simulink model "Katex_FullCar_R2017b_V03"  (R2026a)
settings: Solver=ode1  StopTime=1000  FixedStep=Ts  EnableMultiTasking=on
PostLoadFcn:
  | , if any(exist('dsrtsu_mdlpostloadfcn', 'file') == [2, 3, 6]), try dsrtsu_mdlpostloadfcn('Execute', bdroot); catch fprintf('Error in PostLoadFcn (dsrtsu_mdlpostloadfcn) for model "%s":\n %s\n', bdroot, lasterr); end, end,
  | , if any(exist('dsrtsu_mdlpostloadfcn', 'file') ~= 0), dsrtsu_mdlpostloadfcn('Execute', bdroot); end,
InitFcn:
  | , if any(exist('rtifpga_mdlclblib', 'file') ~= 0), rtifpga_mdlclblib('Init', bdroot); end,
  | 
  | 
  | init
undefined symbols (not defined in the file): locklim_sus, roundN, Ts
libraries: sl_discontinuities x29, simulink_extras x26, simulink x22, mjLib x1
(part 1 of 10)
Description:
  | Standard RTI1401 template.
  | Supported MATLAB version:  R2018b.
settings Model: Tag=RTI1401  DSRTSU_INTERNAL_RTI_VER=510  DSRTSU_INTERNAL_RTI_TYPE=rti1401  RTICANMMDATA=struct('GeneralSetupData',struct('modelroot','C:\Users\USER\Desktop\KATEC_FullCar\simulink','generalsettings',struct('filesettings',struct('destfolder',struct('Name','RTICANMM_FILES','Check',1),'buildfolder',struct('Name','.','Check',1),'AbsDestfolder',struct('Name','C:\Users\USER\Desktop\KATEC_FullCar\simulink\RTICANMM_FILES'),'AbsBuildfolder',struct('Name','C:\Users\USER\Desktop\KATEC_FullCar\simulink'))),'options',struct('addpaths',1,'rmpaths',1,'addtrcexclusion',logical(1),'cannavigator',struct('checkmonitoring',0),'show_usrtrc',0,'use_usrtrc',0),'advanced',struct('options',[1 1 1 1 1 1 1 1 1 1 1 1 1 1 1 1 1 1 1 1 1 1 1 1 1 1 1 1 1 1 1 1 1 1 1 1 1 1 1 1 1 1 1 1 1 1 1 1 1 1 1 1 1 1 1 1 1 1 1 1 1 1 1 1 1 1 1 1 1 1 1 1 1 1 1 1 1 1 1 1 1 1 1 1 1 1 1 1 1 1 1 1 1 1 1 1 1 1 1 1]),'MPSetup',{{}},'modelname','Katex_FullCar_R2017b_V03','block','Katex_FullCar_R2017b_V03'))  DSRTSU_INTERNAL_RTIFLEXRAYCONFIG=110  DSRTSU_INTERNAL_RTIFPGA=110  Creator=KATECH  LastModifiedBy=minsu
settings DataIOCC: SaveFormat=StructureWithTime
settings OptimizationCC: OptimizeBlockIOStorage=off  BufferReuse=off  GlobalBufferReuse=off  ExpressionFolding=off  LocalBlockOutputs=off  OptimizeDataStoreBuffers=off  BusAssignmentInplaceUpdate=off
settings HardwareCC: ProdLargestAtomicInteger=Integer  ProdEndianess=BigEndian  ProdHWDeviceType=Custom Processor->Custom  TargetIntDivRoundTo=Zero  TargetEndianess=BigEndian  TargetHWDeviceType=Custom Processor->Custom
settings ModelReferenceCC: EnableParallelModelReferenceBuilds=on  ParallelModelReferenceMATLABWorkerInit=Load Top Model
settings RTWCC: SystemTargetFile=rti1401.tlc  MakeCommand=make_rti  TemplateMakefile=rti1401.tmf  RTWCompilerOptimization=on  Description=dSPACE DS1401 Hardware Platform
settings STFCustomTargetCC: SystemTargetFile=rti1401.tlc  MultiwordLength=2048.0  ParMdlRefBuildCompliant=on  GRTInterface=off  TRCGenerateLabels=off  AssertionMode=OFF  EnableDataSetStorageNonUI=OFF  TRCGenerateVirtualBlocks=off  TimeScaleFactorNonUI=OPTION_DISABLED  PlatformSelectionPopup=Platform Name  LoadAfterBuild=on  AllowReservedHostServiceNums=off  TRCGenerateParamValues=off  TRCGenerateStates=off  EnableRealTimeTestingNonUI=ON  LoadToFlash=off  CCompilerOptimizationOptsNonUI=USE_DEFAULT  NetworkClientNonUI=OPTION_DISABLED  EnableDataSetStorage=off  InitialSimState=RUN  ExecutionModeNonUI=RTSIM  LoadApplNonUI=ON  BoardName=ds1401  CCompilerOptimizationOptsPopup_=Default  TRCIsOmitVdOn=off  BoardNameNonUI=ds1401  TRCGenerateDerivatives=off  ExecutionMode=real-time  RTICfgSetVer=510.0  TimeScaleFactor=1.0  TRCOnlyGlobals=off  EnableRealTimeTesting=on
settings GRTTargetCC: CompOptLevelCompliant=off  ConcurrentExecutionCompliant=off  CombineOutputUpdateFcns=off  MatFileLogging=off  CPPClassGenCompliant=off
settings ConfigComp: CovMetricSettings=dswe
settings SimscapeCC: SimscapeLogDecimation=1  SimscapeLogType=none  SimscapeNominalValues="[{\"value\":\"1\",\"unit\":\"A\"},{\"value\":\"1\",\"unit\":\"bar\"},{\"value\":\"1\",\"unit\":\"cm^2\"},{\"value\":\"1\",\"unit\":\"cm^3/s\"},{\"value\":\"1\",\"unit\":\"kJ/kg\"},{\"value\":\"1\",\"unit\":\"kW\"},{\"value\":\"1\",\"unit\":\"l\"},{\"value\":\"1\",\"unit\":\"N\"},{\"value\":\"1\",\"unit\":\"N*m\"},{\"value\":\"1\",\"unit\":\"V\"}]"  SimscapeLogDataHistory=5000

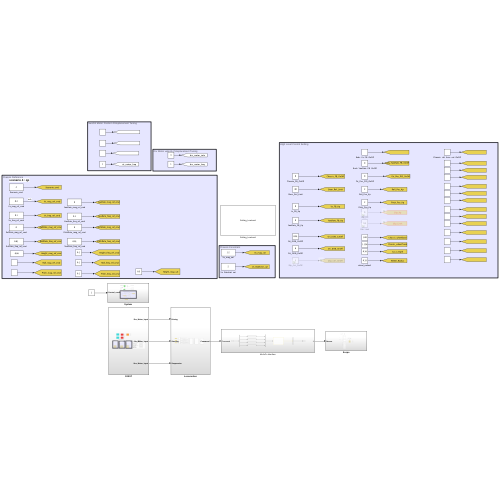
[thumbnail: Simulink's stored preview of the top-level diagram]
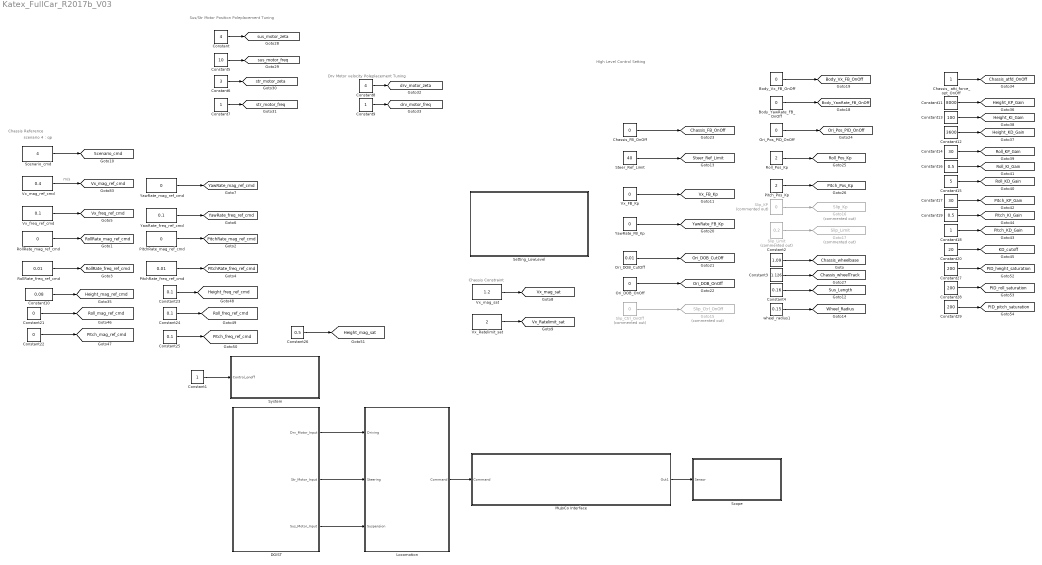
== system Katex_FullCar_R2017b_V03 ==
  note: scenario 4 : qp
  note: Chassis Reference
  note: Drv Motor velocity Poleplacement Tuning
  note: m/s
  note: Chassis Constraint
  note: HIgh Level Control Setting
  note: Sus/Str Motor Position Poleplacement Tuning
  Body_Vx_FB_OnOff : Constant  Value=0
  Body_YawRate_FB_OnOff : Constant  Value=0
  Chassis_ atti_force_opt_OnOff : Constant
  Chassis_FB_OnOff : Constant  Value=0
  Constant : Constant  Value=4
  Constant{1,7,9,18} (4 alike) : Constant
  Constant10 : Constant  Value=0.08
  Constant11 : Constant  Value=8000
  Constant12 : Constant  Value=3600
  Constant13 : Constant  Value=100
  Constant14 : Constant  Value=30
  Constant15 : Constant  Value=5
  Constant16 : Constant  Value=0.5
  Constant17 : Constant  Value=30
  Constant19 : Constant  Value=0.5
  Constant2 : Constant  Value=1.09
  Constant20 : Constant  Value=20
  Constant21 : Constant  Value=0
  Constant22 : Constant  Value=0
  Constant23 : Constant  Value=0.1
  Constant24 : Constant  Value=0.1
  Constant25 : Constant  Value=0.1
  Constant26 : Constant  Value=0.5
  Constant27 : Constant  Value=200
  Constant28 : Constant  Value=200
  Constant29 : Constant  Value=200
  Constant3 : Constant  Value=1.126
  Constant4 : Constant  Value=0.16
  Constant5 : Constant  Value=10
  Constant6 : Constant  Value=3
  Constant8 : Constant  Value=4
  DGIST : Subsystem
  Goto15 : Goto  Commented=on  GotoTag=Slip_Ctrl_OnOff  TagVisibility=global
  Goto16 : Goto  Commented=on  GotoTag=Slip_Kp  TagVisibility=global
  Goto17 : Goto  Commented=on  GotoTag=Slip_Limit  TagVisibility=global
  Locomotion : Subsystem
  MuJoCo Interface : Subsystem
  Ori_DOB_CutOff : Constant  Value=0.01
  Ori_DOB_OnOff : Constant  Value=0
  Ori_Pos_PID_OnOff : Constant  Value=0
  PitchRate_freq_ref_cmd : Constant  Value=0.01
  PitchRate_mag_ref_cmd : Constant  Value=0
  Pitch_Pos_Kp : Constant  Value=2
  RollRate_freq_ref_cmd : Constant  Value=0.01
  RollRate_mag_ref_cmd : Constant  Value=0
  Roll_Pos_Kp : Constant  Value=2
  Scenario_cmd : Constant  Value=4
  Scope : Subsystem
  Setting_LowLevel : Subsystem
      mask Display: disp('Setting_LowLevel');
  Slip_Ctrl_OnOff : Constant  Commented=on  Value=0
  Slip_KP : Constant  Commented=on  Value=0
  Slip_Limit : Constant  Commented=on  Value=0.2
  Steer_Ref_Limit : Constant  Value=40
  System : Subsystem
  Vx_FB_Kp : Constant  Value=0
  Vx_Ratelimit_sat : Constant  Value=2
  Vx_freq_ref_cmd : Constant  Value=0.1
  Vx_mag_ref_cmd : Constant  Value=0.4
  Vx_mag_sat : Constant  Value=1.2
  YawRate_FB_Kp : Constant  Value=0
  YawRate_freq_ref_cmd : Constant  Value=0.1
  YawRate_mag_ref_cmd : Constant  Value=0
  wheel_radius1 : Constant  Value=0.15
  tag scope: Body_Vx_FB_OnOff=global, Body_YawRate_FB_OnOff=global, Chassis_FB_OnOff=global, Chassis_atfd_OnOff=global, Chassis_wheelTrack=global, Chassis_wheelbase=global, Height_KD_Gain=global, Height_KI_Gain=global, Height_KP_Gain=global, Height_freq_ref_cmd=global, Height_mag_ref_cmd=global, Height_mag_sat=global, KD_cutoff=global, Ori_DOB_CutOff=global, Ori_DOB_OnOff=global, Ori_Pos_PID_OnOff=global, PID_height_saturation=global, PID_pitch_saturation=global, PID_roll_saturation=global, PitchRate_freq_ref_cmd=global, PitchRate_mag_ref_cmd=global, Pitch_KD_Gain=global, Pitch_KI_Gain=global, Pitch_KP_Gain=global, Pitch_Pos_Kp=global, Pitch_freq_ref_cmd=global, Pitch_mag_ref_cmd=global, RollRate_freq_ref_cmd=global, RollRate_mag_ref_cmd=global, Roll_KD_Gain=global, Roll_KI_Gain=global, Roll_KP_Gain=global, Roll_Pos_Kp=global, Roll_freq_ref_cmd=global, Roll_mag_ref_cmd=global, Scenario_cmd=global, Steer_Ref_Limit=global, Sus_Length=global, Vx_FB_Kp=global, Vx_Ratelimit_sat=global, Vx_freq_ref_cmd=global, Vx_mag_ref_cmd=global, Vx_mag_sat=global, Wheel_Radius=global, YawRate_FB_Kp=global, YawRate_freq_ref_cmd=global, YawRate_mag_ref_cmd=global, drv_motor_freq=global, drv_motor_zeta=global, str_motor_freq=global, str_motor_zeta=global, sus_motor_freq=global, sus_motor_zeta=global
  wires:
  DGIST/1(Drv_Motor_Input) -> Locomotion/1(Driving)
  DGIST/2(Str_Motor_Input) -> Locomotion/2(Steering)
  MuJoCo Interface/1(Out1) -> Scope/1(Sensor)
  Locomotion/1(Command) -> MuJoCo Interface/1(Command)
  Constant1/1 -> System/1(Control_onoff)
  RollRate_freq_ref_cmd/1 -> [RollRate_freq_ref_cmd]
  YawRate_freq_ref_cmd/1 -> [YawRate_freq_ref_cmd]
  Vx_mag_ref_cmd/1 -> [Vx_mag_ref_cmd]
  RollRate_mag_ref_cmd/1 -> [RollRate_mag_ref_cmd]
  Vx_Ratelimit_sat/1 -> [Vx_Ratelimit_sat]
  Vx_freq_ref_cmd/1 -> [Vx_freq_ref_cmd]
  Scenario_cmd/1 -> [Scenario_cmd]
  PitchRate_mag_ref_cmd/1 -> [PitchRate_mag_ref_cmd]
  Vx_mag_sat/1 -> [Vx_mag_sat]
  PitchRate_freq_ref_cmd/1 -> [PitchRate_freq_ref_cmd]
  YawRate_mag_ref_cmd/1 -> [YawRate_mag_ref_cmd]
  Constant2/1 -> [Chassis_wheelbase]
  Slip_Ctrl_OnOff/1 -> Goto15/1
  Body_YawRate_FB_OnOff/1 -> [Body_YawRate_FB_OnOff]
  Vx_FB_Kp/1 -> [Vx_FB_Kp]
  Ori_Pos_PID_OnOff/1 -> [Ori_Pos_PID_OnOff]
  Slip_KP/1 -> Goto16/1
  YawRate_FB_Kp/1 -> [YawRate_FB_Kp]
  Roll_Pos_Kp/1 -> [Roll_Pos_Kp]
  Pitch_Pos_Kp/1 -> [Pitch_Pos_Kp]
  Constant4/1 -> [Sus_Length]
  Slip_Limit/1 -> Goto17/1
  Ori_DOB_OnOff/1 -> [Ori_DOB_OnOff]
  Ori_DOB_CutOff/1 -> [Ori_DOB_CutOff]
  Steer_Ref_Limit/1 -> [Steer_Ref_Limit]
  Chassis_FB_OnOff/1 -> [Chassis_FB_OnOff]
  wheel_radius1/1 -> [Wheel_Radius]
  Body_Vx_FB_OnOff/1 -> [Body_Vx_FB_OnOff]
  Constant3/1 -> [Chassis_wheelTrack]
  Constant/1 -> [sus_motor_zeta]
  Constant5/1 -> [sus_motor_freq]
  Constant7/1 -> [str_motor_freq]
  Constant6/1 -> [str_motor_zeta]
  Constant8/1 -> [drv_motor_zeta]
  Constant9/1 -> [drv_motor_freq]
  Chassis_ atti_force_opt_OnOff/1 -> [Chassis_atfd_OnOff]
  DGIST/3(Sus_Motor_Input) -> Locomotion/3(Suspension)
  Constant11/1 -> [Height_KP_Gain]
  Constant12/1 -> [Height_KD_Gain]
  Constant13/1 -> [Height_KI_Gain]
  Constant14/1 -> [Roll_KP_Gain]
  Constant16/1 -> [Roll_KI_Gain]
  Constant15/1 -> [Roll_KD_Gain]
  Constant17/1 -> [Pitch_KP_Gain]
  Constant19/1 -> [Pitch_KI_Gain]
  Constant18/1 -> [Pitch_KD_Gain]
  Constant20/1 -> [KD_cutoff]
  Constant10/1 -> [Height_mag_ref_cmd]
  Constant21/1 -> [Roll_mag_ref_cmd]
  Constant22/1 -> [Pitch_mag_ref_cmd]
  Constant23/1 -> [Height_freq_ref_cmd]
  Constant24/1 -> [Roll_freq_ref_cmd]
  Constant25/1 -> [Pitch_freq_ref_cmd]
  Constant26/1 -> [Height_mag_sat]
  Constant27/1 -> [PID_height_saturation]
  Constant28/1 -> [PID_roll_saturation]
  Constant29/1 -> [PID_pitch_saturation]

== system Katex_FullCar_R2017b_V03/DGIST ==
  note: Str Plant Input
      |
      | Motor Input => cnt or Target Torque
  note: Plant Input에 연결시키면 됨
  note: Hardware ActVal에서 변환 필요
  note: Drive Plant Input
      |
      | Motor Input => RPM or Target Torque
  note: Motor Driver
      | vel은 RPM / Pos cnt / Torque mA로 나옴(모터 상수이용해서 Nm 교체 필요)
      | Dri__ , Sus__, Str__ , 빈칸에는 FL,FR,RL,RR 작성 필요
      | 각 Controller에 measure 자리에 집어 넣어야함
      |
      | Drive Wheel단 Load rad/s measure
      | Drive wheel단 Load Nm measure
      |
      | Suspension Load deg measure
      | Suspension Load rad/s measure
      | Suspension Load Nm measure
      | Suspension Load rad measure(highlevel)
      |
      | Steer Load deg measure
      | Steer Load Nm measure
      |
      | IMU RollRate LPF measure
      | IMU PitchRate LPF measure
      | IMU Roll angle LPF measure
      | IMU Pitch angle LPF measure
      |
      | 후륜 Load rad/s를 가지고 Vx setting
      | slip ratio도 해당꺼로 계산 필요
  note: Sus Plant Input
      |
      | Motor Input => cnt or RPM
      | Not Yet Torque Mode
  Attitude&Force distribution opt : Subsystem
      mask Display: disp('Force Distribution Opt');
  Attitude_reference_generator : Subsystem
      mask Display: disp('_Reference_Generator')
  Subsystem : Subsystem
      mask Display: disp('Dri_actRPM_2_Load[Rad/s]');
  Subsystem1 : Subsystem
      mask Display: disp('Dri_actTorque_2_Load[Nm]');
  Subsystem10 : Subsystem  Commented=on
      mask Display: disp('Imu_Pitch_LPF');
  Subsystem11 : Subsystem
      mask Display: disp('Sus_actPos_2_Load[rad]');
  Subsystem12 : Subsystem  Commented=on
      mask Display: disp('Imu_RollRate_LPF');
  Subsystem13 : Subsystem
      mask Display: disp('Dri_ref(m/s)_2_motor(rad/s)');
  Subsystem2 : Subsystem
      mask Display: disp('Sus_actPos_2_Load[deg]');
  Subsystem3 : Subsystem
      mask Display: disp('Sus_actVel_2_Load[rad/s]');
  Subsystem4 : Subsystem
      mask Display: disp('Sus_actTorque_2_Load[Nm]');
  Subsystem5 : Subsystem
      mask Display: disp('Str_actTorque_2_Load[Nm]');
  Subsystem6 : Subsystem
      mask Display: disp('Str_actPos_2_Load[deg]');
  Subsystem7 : Subsystem  Commented=on
      mask Display: disp('Imu_PitchRate_LPF');
  Subsystem8 : Subsystem  Commented=on
      mask Display: disp('Imu_RollRate_LPF');
  Subsystem9 : Subsystem  Commented=on
      mask Display: disp('Imu_Roll_LPF');
  _High_Level_Ctrl : Subsystem
      mask Display: disp('High Level Controller');
  _Low_Level_Ctrl : Subsystem
      mask Display: disp('Low Level Controller')
  _Reference_Generator : Subsystem
      mask Display: disp('_Reference_Generator')
  Drv_Motor_Input : Outport  VectorParamsAs1DForOutWhenUnconnected=off
  Str_Motor_Input : Outport  Port=2  VectorParamsAs1DForOutWhenUnconnected=off
  Sus_Motor_Input : Outport  Port=3  VectorParamsAs1DForOutWhenUnconnected=off
  wires:
  _High_Level_Ctrl/2(Str_Load_Vel_Ref) -> _Low_Level_Ctrl/2(In2)  "Str_Load_Vel_Ref"
  _Low_Level_Ctrl/2(Out2) -> Str_Motor_Input/1
  _Low_Level_Ctrl/1(Out1) -> Drv_Motor_Input/1
  _Low_Level_Ctrl/3(Out3) -> Sus_Motor_Input/1
  Attitude_reference_generator/1(Out1) -> Attitude&Force distribution opt/1(u)
  Attitude&Force distribution opt/2(Desired_sus_torque[4X1]) -> _Low_Level_Ctrl/3(In3)  "Sus_Torque_Ref"
  Attitude&Force distribution opt/1(vx[m/s]) -> _Low_Level_Ctrl/1(In1)

== system Katex_FullCar_R2017b_V03/Locomotion ==
  Driving : Inport
  Steering : Inport  Port=2
  Suspension : Inport  Port=3
  Branch : Subsystem
  Conditioning : Subsystem
  If Action Subsystem : Subsystem  TreatAsAtomicUnit=on
  If Action Subsystem1 : Subsystem  TreatAsAtomicUnit=on
  If Action Subsystem2 : Subsystem  TreatAsAtomicUnit=on
  If Action Subsystem3 : Subsystem  TreatAsAtomicUnit=on
  If Action Subsystem4 : Subsystem  TreatAsAtomicUnit=on
  If Action Subsystem5 : Subsystem  TreatAsAtomicUnit=on
  If1 : If  IfExpression=u1 == 1  ElseIfExpressions=u1 == 2
  If2 : If  IfExpression=u1 == 0||u1==1  ElseIfExpressions=u1 == 2
  If3 : If  IfExpression=u1 == 0||u1==1  ElseIfExpressions=u1 == 2
  Initialization : Subsystem
  Command : Outport  VectorParamsAs1DForOutWhenUnconnected=off
  wires:
  Branch/3(RL) -> Initialization/3(RLin)
  Branch/4(RR) -> Initialization/4(RRin)
  Branch/2(FR) -> Initialization/2(FRin)
  Conditioning/3(Str_angle) -> Branch/3(str_angref_deg)
  Conditioning/2(Drv_torque) -> Branch/2(drv_tqref_Nm)
  Conditioning/5(Sus_angle) -> Branch/5(sus_angref_deg)
  Conditioning/4(Str_torque) -> Branch/4(str_tqref_Nm)
  Conditioning/1(Drv_velocity) -> Branch/1(drv_velref_mps)
  Branch/1(FL) -> Initialization/1(FLin)
  Initialization/1(Controller) -> Command/1
  Driving/1 -> If Action Subsystem/1(In1), If Action Subsystem1/1(Driving)
  [Dri_Motor_Mode] -> If1/1
  If1/1 -> If Action Subsystem/Action
  If Action Subsystem/1(CMD_DRV_VELOCITY) -> Conditioning/1(CMD_DRV_VELOCITY)
  If Action Subsystem1/1(CMD_DRV_VELOCITY) -> Conditioning/2(CMD_DRV_TORQUE)
  If1/2 -> If Action Subsystem1/Action
  Steering/1 -> If Action Subsystem3/1(Driving), If Action Subsystem2/1(In1)
  If2/2 -> If Action Subsystem3/Action
  If2/1 -> If Action Subsystem2/Action
  If Action Subsystem2/1(CMD_DRV_VELOCITY) -> Conditioning/3(CMD_STR_ANGLE)
  If Action Subsystem3/1(CMD_DRV_VELOCITY) -> Conditioning/4(CMD_STR_TORQUE)
  [Str_Motor_Mode] -> If2/1
  If3/2 -> If Action Subsystem5/Action
  If3/1 -> If Action Subsystem4/Action
  [Sus_Motor_Mode] -> If3/1
  Suspension/1 -> If Action Subsystem5/1(Driving), If Action Subsystem4/1(Suspension)
  If Action Subsystem4/1(CMD_DRV_VELOCITY) -> Conditioning/5(CMD_SUS_ANGLE)
  If Action Subsystem5/1(CMD_DRV_VELOCITY) -> Conditioning/6(CMD_SUS_TORQUE)
  Conditioning/6(Sus_torque) -> Branch/6(sus_tqref_Nm)

== system Katex_FullCar_R2017b_V03/MuJoCo Interface ==
  Command : Inport
  Bus Creator : BusCreator  Inputs=4
  Bus Selector : BusSelector  OutputSignals=torque_sensor_FL,torque_sensor_FR,torque_sensor_RL,torque_sensor_RR,imu_acc,imu_gyro,trunk_vel,trunk_angvel,trunk_pos,trunk_ang,ENC_FL_sus,ENC_FL_steer,ENC_FL_drive,ENC_FR_sus,ENC_FR_steer,ENC_FR_drive,ENC_RL_sus,ENC_RL_steer,ENC_RL_drive,ENC_RR_sus,ENC_RR_steer,ENC_RR_drive,touch_FL,grf_seonsor_FL,touch_FR,grf_seonsor_FR,touch_RL,grf_seonsor_RL,touch_RR,grf_seonsor_RR,Vel_FL_sus,Vel_FR_sus,Vel_RL_sus,Vel_RR_sus,Vel_FL_steer,Vel_FR_steer,Vel_RL_steer,Vel_RR_steer,Vel_FL_drv,Vel_FR_drv,Vel_RL_drv,Vel_RR_drv,FL_sus_actuator_torque,FR_sus_actuator_torque,RL_sus_actuator_torque,RR_sus_actuator_torque  OutputAsBus=on
  Bus Selector1 : BusSelector  OutputSignals=FL,FR,RL,RR
  FL_Motor_Control : Subsystem
  FR_Motor_Control : Subsystem
  MuJoCo Plant : mjLib/MuJoCo Plant  controlBus=[]  sensorBus=mj_bus_sensor_7979902499018342666  controlLength=[]  sensorLength=[]  rgbLength=[]  depthLength=[]  sampleTime=0.001  xmlFileRel=/home/minsu/MuJoCo_Rover_CTRL/model/mcl_rover/scene_terrain.xml  xmlFile=/home/minsu/MuJoCo_Rover_CTRL/model/mcl_rover/scene_terrain.xml  renderingType=Global  vsync=off  visualFPS=60  zoomLevel=1  znear=0.03  zfar=150  cameraSampleTime=0.001  rgbOutOption=on  depthOutOption=on  controlInterfaceType=Vector
      settings: SourceProductName=MuJoCo Simulator
  RL_Motor_Control : Subsystem
  RR_Motor_Control : Subsystem
  Out1 : Outport
  wires:
  RL_Motor_Control/1(Out2) -> Bus Creator/3  "RL"
  RR_Motor_Control/1(Out2) -> Bus Creator/4  "RR"
  Bus Creator/1 -> MuJoCo Plant/1
  FR_Motor_Control/1(Out2) -> Bus Creator/2  "FR"
  Command/1 -> Bus Selector1/1
  Bus Selector1/1 -> FL_Motor_Control/1(In1)  "<FL>"
  Bus Selector1/2 -> FR_Motor_Control/1(In1)  "<FR>"
  Bus Selector1/3 -> RL_Motor_Control/1(In1)  "<RL>"
  Bus Selector1/4 -> RR_Motor_Control/1(In1)  "<RR>"
  MuJoCo Plant/1 -> Bus Selector/1
  Bus Selector/1 -> Out1/1
  FL_Motor_Control/1(Out2) -> Bus Creator/1  "FL"

== system Katex_FullCar_R2017b_V03/Scope ==
  Sensor : Inport
  Body_PitchRate_ref : Scope
      settings: DataLoggingVariableName=ScopeData4
  Body_RollRate_ref : Scope
      settings: DataLoggingVariableName=ScopeData3
  Body_Vx_ref : Scope
  Body_YawRate_ref : Scope
      settings: DataLoggingVariableName=ScopeData2
  Controlword_cmd : Scope
      settings: DataLoggingVariableName=ScopeData28
  Demux : Demux  Outputs=2
  FL : Subsystem
  FR : Subsystem
  IMU : Subsystem
  Initialization_Status : Subsystem
  NMT_NodeID : Scope
      settings: DataLoggingVariableName=ScopeData27
  NMT_cmd : Scope
  RL : Subsystem
  RR : Subsystem
  TOUCH : Subsystem
  Torque_sensor : Scope  NumInputPorts=4
      settings: ActiveDisplayYMinimum=-8.5141737367185648  ActiveDisplayYMaximum=2.7458236474698614  DataLoggingVariableName=ScopeData96
  Trunk : Subsystem
  wires:
  [NMT] -> Demux/1
  Sensor/1 -> RR/1(Plant), TOUCH/1(Sensor), Trunk/1(Sensor), IMU/1(In1), RL/1(Plant), FR/1(Plant), FL/1(Plant)
  [Controller] -> FL/2(Controller), FR/2(Controller), RL/2(Controller), RR/2(Controller)
  Demux/1 -> NMT_cmd/1
  Demux/2 -> NMT_NodeID/1
  [controlword_cmd] -> Controlword_cmd/1
  [Body_Pitch_deg_scope] -> Body_PitchRate_ref/1
  [Body_Roll_deg_scope] -> Body_RollRate_ref/1
  [Body_Yawrate_degps_scope] -> Body_YawRate_ref/1
  [Body_vx_mps_scope] -> Body_Vx_ref/1
  [RL_sus_torque] -> Torque_sensor/3  "RL"
  [RR_Sus_torque] -> Torque_sensor/4  "RR"
  [FR_sus_torque] -> Torque_sensor/2  "FR"
  [FL_sus_torque] -> Torque_sensor/1  "FL"

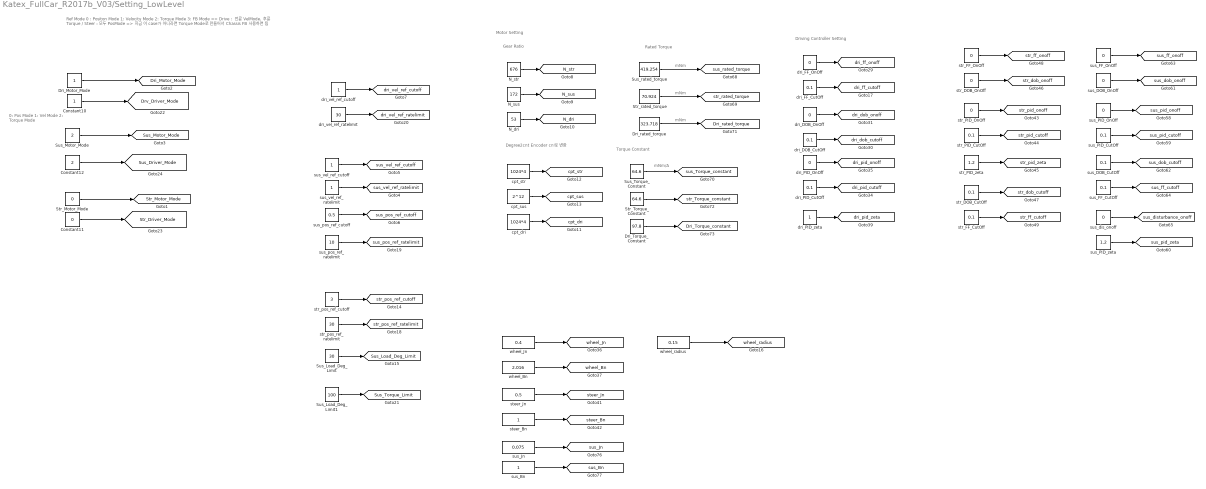
== system Katex_FullCar_R2017b_V03/Setting_LowLevel ==
  note: Motor Setting
  note: Ref Mode
      |
      | 0 : Positon Mode
      | 1: Velocity Mode
      | 2: Torque Mode
      | 3: FB Mode => Drive : 전륜 VelMode, 후륜 Torque / Steer : 모두 PosMode => 지금 이 case가 아니라면 Torque Mode로 만들어서 Chassis FB 사용하면 됨
  note: mNm
  note: Rated Torque
  note: Gear Ratio
  note: Degree2cnt
      | Encoder cnt로 변환
  note: mNm
  note: mNm
  note: Torque Constant
  note: mNm/A
  note: Driving Controller Setting
  note: 0: Pos Mode
      | 1: Vel Mode
      | 2: Torque Mode
  Constant10 : Constant
  Constant11 : Constant  Value=0
  Constant12 : Constant  Value=2
  Dri_Motor_Mode : Constant
  Dri_Torque_Constant : Constant  Value=97.8
  Dri_rated_torque : Constant  Value=323.718
  N_dri : Constant  Value=53
  N_str : Constant  Value=676
  N_sus : Constant  Value=172
  Str_Motor_Mode : Constant  Value=0
  Str_Torque_Constant : Constant  Value=64.6
  Str_rated_torque : Constant  Value=70.924
  Sus_Load_Deg_Limit : Constant  Value=30
  Sus_Load_Deg_Limit1 : Constant  Value=100
  Sus_Motor_Mode : Constant  Value=2
  Sus_Torque_Constant : Constant  Value=64.6
  Sus_rated_torque : Constant  Value=419.254
  cpt_dri : Constant  Value=1024*4
  cpt_str : Constant  Value=1024*4
  cpt_sus : Constant  Value=2^12
  dri_DOB_CutOff : Constant  Value=0.1
  dri_DOB_OnOff : Constant  Value=0
  dri_FF_CutOff : Constant  Value=0.1
  dri_FF_OnOff : Constant  Value=0
  dri_PID_CutOff : Constant  Value=0.1
  dri_PID_OnOff : Constant  Value=0
  dri_PID_zeta : Constant
  dri_vel_ref_cutoff : Constant
  dri_vel_ref_ratelimit : Constant  Value=30
  steer_Bn : Constant
  steer_Jn : Constant  Value=0.5
  str_DOB_CutOff : Constant  Value=0.1
  str_DOB_OnOff : Constant  Value=0
  str_FF_CutOff : Constant  Value=0.1
  str_FF_OnOff : Constant  Value=0
  str_PID_CutOff : Constant  Value=0.1
  str_PID_OnOff : Constant  Value=0
  str_PID_zeta : Constant  Value=1.2
  str_pos_ref_cutoff : Constant  Value=3
  str_pos_ref_ratelimit : Constant  Value=30
  sus_Bn : Constant
  sus_DOB_CutOff : Constant  Value=0.1
  sus_DOB_OnOff : Constant  Value=0
  sus_FF_CutOff : Constant  Value=0.1
  sus_FF_OnOff : Constant  Value=0
  sus_Jn : Constant  Value=0.075
  sus_PID_CutOff : Constant  Value=0.1
  sus_PID_OnOff : Constant  Value=0
  sus_PID_zeta : Constant  Value=1.2
  sus_dis_onoff : Constant  Value=0
  sus_pos_ref_cutoff : Constant  Value=0.5
  sus_pos_ref_ratelimit : Constant  Value=10
  sus_vel_ref_cutoff : Constant
  sus_vel_ref_ratelimit : Constant
  wheel_Bn : Constant  Value=2.016
  wheel_Jn : Constant  Value=0.4
  wheel_radius : Constant  Value=0.15
  tag scope: Dri_Motor_Mode=global, Dri_Torque_constant=global, Dri_rated_torque=global, Drv_Driver_Mode=global, N_dri=global, N_str=global, N_sus=global, Str_Driver_Mode=global, Str_Motor_Mode=global, Sus_Driver_Mode=global, Sus_Load_Deg_Limit=global, Sus_Motor_Mode=global, Sus_Torque_Limit=global, cpt_dri=global, cpt_str=global, cpt_sus=global, dri_dob_cutoff=global, dri_dob_onoff=global, dri_ff_cutoff=global, dri_ff_onoff=global, dri_pid_cutoff=global, dri_pid_onoff=global, dri_pid_zeta=global, dri_vel_ref_cutoff=global, dri_vel_ref_ratelimit=global, steer_Bn=global, steer_Jn=global, str_Torque_constant=global, str_dob_cutoff=global, str_dob_onoff=global, str_ff_cutoff=global, str_ff_onoff=global, str_pid_cutoff=global, str_pid_onoff=global, str_pid_zeta=global, str_pos_ref_cutoff=global, str_pos_ref_ratelimit=global, str_rated_torque=global, sus_Bn=global, sus_Jn=global, sus_Torque_constant=global, sus_disturbance_onoff=global, sus_dob_cutoff=global, sus_dob_onoff=global, sus_ff_cutoff=global, sus_ff_onoff=global, sus_pid_cutoff=global, sus_pid_onoff=global, sus_pid_zeta=global, sus_pos_ref_cutoff=global, sus_pos_ref_ratelimit=global, sus_rated_torque=global, sus_vel_ref_cutoff=global, sus_vel_ref_ratelimit=global, wheel_Bn=global, wheel_Jn=global, wheel_radius=global
  wires:
  Dri_Motor_Mode/1 -> [Dri_Motor_Mode]
  Sus_Motor_Mode/1 -> [Sus_Motor_Mode]
  Str_Motor_Mode/1 -> [Str_Motor_Mode]
  dri_vel_ref_cutoff/1 -> [dri_vel_ref_cutoff]
  dri_vel_ref_ratelimit/1 -> [dri_vel_ref_ratelimit]
  Str_rated_torque/1 -> [str_rated_torque]
  N_str/1 -> [N_str]
  N_dri/1 -> [N_dri]
  cpt_str/1 -> [cpt_str]
  cpt_dri/1 -> [cpt_dri]
  Sus_rated_torque/1 -> [sus_rated_torque]
  Dri_rated_torque/1 -> [Dri_rated_torque]
  N_sus/1 -> [N_sus]
  cpt_sus/1 -> [cpt_sus]
  sus_vel_ref_ratelimit/1 -> [sus_vel_ref_ratelimit]
  sus_vel_ref_cutoff/1 -> [sus_vel_ref_cutoff]
  sus_pos_ref_cutoff/1 -> [sus_pos_ref_cutoff]
  sus_pos_ref_ratelimit/1 -> [sus_pos_ref_ratelimit]
  str_pos_ref_cutoff/1 -> [str_pos_ref_cutoff]
  str_pos_ref_ratelimit/1 -> [str_pos_ref_ratelimit]
  Sus_Torque_Constant/1 -> [sus_Torque_constant]
  Str_Torque_Constant/1 -> [str_Torque_constant]
  sus_Bn/1 -> [sus_Bn]
  steer_Bn/1 -> [steer_Bn]
  steer_Jn/1 -> [steer_Jn]
  sus_Jn/1 -> [sus_Jn]
  wheel_Jn/1 -> [wheel_Jn]
  wheel_Bn/1 -> [wheel_Bn]
  Dri_Torque_Constant/1 -> [Dri_Torque_constant]
  str_PID_OnOff/1 -> [str_pid_onoff]
  str_PID_zeta/1 -> [str_pid_zeta]
  sus_PID_CutOff/1 -> [sus_pid_cutoff]
  dri_FF_CutOff/1 -> [dri_ff_cutoff]
  dri_PID_zeta/1 -> [dri_pid_zeta]
  sus_FF_OnOff/1 -> [sus_ff_onoff]
  str_DOB_CutOff/1 -> [str_dob_cutoff]
  str_DOB_OnOff/1 -> [str_dob_onoff]
  str_FF_OnOff/1 -> [str_ff_onoff]
  dri_PID_CutOff/1 -> [dri_pid_cutoff]
  dri_DOB_OnOff/1 -> [dri_dob_onoff]
  dri_FF_OnOff/1 -> [dri_ff_onoff]
  dri_PID_OnOff/1 -> [dri_pid_onoff]
  sus_FF_CutOff/1 -> [sus_ff_cutoff]
  dri_DOB_CutOff/1 -> [dri_dob_cutoff]
  sus_PID_zeta/1 -> [sus_pid_zeta]
  str_PID_CutOff/1 -> [str_pid_cutoff]
  sus_PID_OnOff/1 -> [sus_pid_onoff]
  sus_dis_onoff/1 -> [sus_disturbance_onoff]
  str_FF_CutOff/1 -> [str_ff_cutoff]
  sus_DOB_CutOff/1 -> [sus_dob_cutoff]
  sus_DOB_OnOff/1 -> [sus_dob_onoff]
  Sus_Load_Deg_Limit/1 -> [Sus_Load_Deg_Limit]
  wheel_radius/1 -> [wheel_radius]
  Sus_Load_Deg_Limit1/1 -> [Sus_Torque_Limit]
  Constant10/1 -> [Drv_Driver_Mode]
  Constant11/1 -> [Str_Driver_Mode]
  Constant12/1 -> [Sus_Driver_Mode]

== system Katex_FullCar_R2017b_V03/System ==
  note: 0x01 [1] - Operational
      | 0x80 [128] - Pre-operational
      | 0x81 [129] - Power reset
  note: 0x06 [6] - Shutdown
      | 0x0F [15] - Enable
  note: 0x09 [9] - CSV
      | 0x0A [10] - CST
  note: Control Time
  Control_onoff : Inport
  Add : Sum
  Constant : Constant
  Data_Logging : Constant  Value=2
  Delay1 : Delay  DelayLength=1  InitialCondition=0
  Gain : Gain  Gain=Ts
  MNT : Constant  Description=|  Value=128  SampleTime=Ts
      | 0x01 [1] - Operational
      | 0x80 [128] - Pre-operational
      | 0x81 [129] - Power reset
  Mux : Mux  Inputs=2
  Product : Product
  _MNT_ID : Constant  Value=0  SampleTime=Ts
  drv_opmode : Constant  Description=|  Value=9  SampleTime=Ts
      | 0x06 [6] - Shutdown
      | 0x0F [15] - Enable
  tag scope: Data_Logging=global, Local_Time=global, NMT=global, controlword_cmd=global, ctrl_onoff=global, drv_opmode_cmd=global
  wires:
  _MNT_ID/1 -> Mux/2
  MNT/1 -> Mux/1
  Constant/1 -> [controlword_cmd]
  Mux/1 -> [NMT]
  drv_opmode/1 -> [drv_opmode_cmd]
  Control_onoff/1 -> [ctrl_onoff], Product/1, Gain/1
  Gain/1 -> Add/1
  Delay1/1 -> Add/2
  Add/1 -> Product/2
  Product/1 -> [Local_Time], Delay1/1
  Data_Logging/1 -> [Data_Logging]

== system Katex_FullCar_R2017b_V03/DGIST/Attitude&Force distribution opt ==
  note: Block에 대한 설명
      |
      | Input
      | - Chassis Body State( Height , Roll, Pitch )
      |
      | Output
      | - Sus Torque (FL,FR,RL,RR)
  u : Inport
  "AX=b, QP" : Subsystem
  Demux{,1..4} (5 alike) : Demux
  "Desired Height, Roll, Pitch Caculate" : Subsystem
  Desired Wrench(PID) : Subsystem
  Desired wrench : Scope
      settings: ActiveDisplayYMinimum=-250  ActiveDisplayYMaximum=250  DataLoggingVariableName=ScopeData84
  Fz[N] : Scope  NumInputPorts=4
      settings: ActiveDisplayYMinimum=-12.500000000000014  ActiveDisplayYMaximum=112.5  DataLoggingVariableName=ScopeData79
  GRF to Joint Torque : Subsystem
  Gain : Gain
  Mux : Mux
  Mux1 : Mux
  Product : Product
  Torque_tracking : Scope  NumInputPorts=5
      settings: ActiveDisplayYMinimum=-16.329999337859736  ActiveDisplayYMaximum=3.6699999264288596  DataLoggingVariableName=ScopeData82
  vx[m/s] : Outport
  Desired_sus_torque[4X1] : Outport  Port=2
  wires:
  u/1 -> "Desired Height, Roll, Pitch Caculate"/1(u)  "Desired Attitude Reference [3X1]"
  "Desired Height, Roll, Pitch Caculate"/1(Desired Attitude Error [3X1]) -> Desired Wrench(PID)/1(Error)
  Desired Wrench(PID)/1(Desired Wrench [3X1]) -> Desired wrench/1, "AX=b, QP"/1(u)
  [AngRoll_deg] -> "Desired Height, Roll, Pitch Caculate"/2(Roll)
  [AngPitch_deg] -> "Desired Height, Roll, Pitch Caculate"/3(Pitch)
  [RRsus_ang_deg] -> Mux/4
  [FLsus_ang_deg] -> Mux/1
  [FRsus_ang_deg] -> Mux/2
  [RLsus_ang_deg] -> Mux/3
  Mux/1 -> [sus_angle_set]
  [sus_angle_set] -> Demux/1
  Demux/1 -> "Desired Height, Roll, Pitch Caculate"/4(Sus_Ang_FL)
  Demux/2 -> "Desired Height, Roll, Pitch Caculate"/5(Sus_Ang_FR)
  Demux/3 -> "Desired Height, Roll, Pitch Caculate"/6(Sus_Ang_RL)
  Demux/4 -> "Desired Height, Roll, Pitch Caculate"/7(Sus_Ang_RR)
  [sus_angle_set] -> Demux1/1
  Demux1/4 -> "AX=b, QP"/5(In5)
  Demux1/3 -> "AX=b, QP"/4(In4)
  Demux1/2 -> "AX=b, QP"/3(In3)
  Demux1/1 -> "AX=b, QP"/2(In2)
  Demux2/4 -> GRF to Joint Torque/5(In5)
  [sus_angle_set] -> Demux2/1
  Demux2/1 -> GRF to Joint Torque/2(In2)
  Demux2/3 -> GRF to Joint Torque/4(In4)
  Demux2/2 -> GRF to Joint Torque/3(In3)
  "AX=b, QP"/1(Desired Fz [4X1]) -> Demux3/1, GRF to Joint Torque/1(In1)
  [Chassis_atfd_OnOff] -> Product/1
  GRF to Joint Torque/1(Desired_sus_torque[4X1]) -> Gain/1
  Product/1 -> Desired_sus_torque[4X1]/1
  Gain/1 -> Demux4/1, Product/2
  [FL_sus_torque] -> Torque_tracking/5  "sensor"
  Mux1/1 -> vx[m/s]/1
  "Desired Height, Roll, Pitch Caculate"/2(vx[m/s]) -> Mux1/4, Mux1/3, Mux1/2, Mux1/1
  Demux3/1 -> Fz[N]/1  "Fz_FL"
  Demux3/2 -> Fz[N]/2  "Fz_FR"
  Demux3/3 -> Fz[N]/3  "Fz_RL"
  Demux3/4 -> Fz[N]/4  "Fz_RR"
  Demux4/4 -> Torque_tracking/4  "T_RR"
  Demux4/3 -> Torque_tracking/3  "T_RL"
  Demux4/2 -> Torque_tracking/2  "T_FR"
  Demux4/1 -> Torque_tracking/1  "T_FL"

== system Katex_FullCar_R2017b_V03/DGIST/Attitude_reference_generator ==
  note: output
      |
      | Height
      | Roll
      | Pitch
      | vx
  Attitude Profile : Subsystem
      mask Display: disp('Attitude Profile');
  Demux : Demux
  Height Tracking : Scope  NumInputPorts=2
      settings: ActiveDisplayYMinimum=-0.020889278905612721  ActiveDisplayYMaximum=0.15635193995799737  DataLoggingVariableName=ScopeData85
  MATLAB Function : MATLAB Function  TreatAsAtomicUnit=on
  Mux : Mux
  Pitch Tracking : Scope  NumInputPorts=2
      settings: ActiveDisplayYMinimum=-12.512307042428906  ActiveDisplayYMaximum=12.612495042660052  DataLoggingVariableName=ScopeData87
  Roll Tracking : Scope  NumInputPorts=2
      settings: ActiveDisplayYMinimum=-12.740045378002952  ActiveDisplayYMaximum=12.695649778168629  DataLoggingVariableName=ScopeData86
  Scope : Scope
      settings: DataLoggingVariableName=ScopeData2
  Scope1 : Scope
      settings: DataLoggingVariableName=ScopeData88
  Out1 : Outport
  wires:
  [Local_Time] -> Scope/1
  Attitude Profile/1(Ref1_Output) -> Demux/1, Out1/1
  Demux/1 -> Height Tracking/1  "ref"
  Demux/2 -> Roll Tracking/1  "ref"
  Demux/3 -> Pitch Tracking/1  "ref"
  [AngRoll_deg] -> Roll Tracking/2  "sensor"
  [AngPitch_deg] -> Pitch Tracking/2  "sensor"
  Mux/1 -> [sus_angle_set]
  [RLsus_ang_deg] -> Mux/3
  [FRsus_ang_deg] -> Mux/2
  [FLsus_ang_deg] -> Mux/1
  [RRsus_ang_deg] -> Mux/4
  [sus_angle_set] -> MATLAB Function/1(u)
  MATLAB Function/1(y) -> Height Tracking/2  "sensor"
  Demux/4 -> Scope1/1

== system Katex_FullCar_R2017b_V03/DGIST/Subsystem ==
  In1 : Inport
  Product : Product  Inputs=*/
  rpm2rad2 : Gain  Gain=2*pi/60
  Out1 : Outport
  wires:
  In1/1 -> rpm2rad2/1  "rpm"
  [N_dri] -> Product/2
  Product/1 -> Out1/1  "Load (rad/s)"
  rpm2rad2/1 -> Product/1  "rad/s"

== system Katex_FullCar_R2017b_V03/DGIST/Subsystem1 ==
  note: A
  note: mNm
  note: mNm/A
  note: Motor Nm
  In1 : Inport
  Divide2 : Product  Inputs=**
  Divide6 : Product  Inputs=**
  Torque Constant1 : Gain  Gain=0.001
  mA2A : Gain  Gain=0.001
  Out2 : Outport
  wires:
  In1/1 -> mA2A/1
  [N_dri] -> Divide2/2
  mA2A/1 -> Divide6/2
  [Dri_Torque_constant] -> Divide6/1
  Torque Constant1/1 -> Divide2/1
  Divide6/1 -> Torque Constant1/1
  Divide2/1 -> Out2/1  "Load[Nm]"

== system Katex_FullCar_R2017b_V03/DGIST/Subsystem10 ==
  In : Inport
  LPF : Subsystem
  Out : Outport
  wires:
  In/1 -> LPF/1(In)
  LPF/1(Out) -> Out/1

== system Katex_FullCar_R2017b_V03/DGIST/Subsystem11 ==
  note: deg motor
  note: cnt
  note: deg load
  In1 : Inport
  Constant3 : Constant  Value=360
  Product3 : Product  Inputs=*/
  Product4 : Product  Inputs=**
  Product5 : Product  Inputs=*/
  deg2rad : Gain  Gain=pi/180
  Out1 : Outport
  wires:
  Constant3/1 -> Product3/1
  Product3/1 -> Product4/2
  Product5/1 -> deg2rad/1
  [N_sus] -> Product5/2
  Product4/1 -> Product5/1
  [cpt_sus] -> Product3/2
  In1/1 -> Product4/1
  deg2rad/1 -> Out1/1

== system Katex_FullCar_R2017b_V03/DGIST/Subsystem12 ==
  In : Inport
  LPF : Subsystem
  Out : Outport
  wires:
  In/1 -> LPF/1(In)
  LPF/1(Out) -> Out/1

== system Katex_FullCar_R2017b_V03/DGIST/Subsystem13 ==
  In1 : Inport
  Product : Product  Inputs=*/
  Out1 : Outport
  wires:
  In1/1 -> Product/1  "m/s"
  Product/1 -> Out1/1  "Load (rad/s)"
  [wheel_radius] -> Product/2

== system Katex_FullCar_R2017b_V03/DGIST/Subsystem2 ==
  note: deg load
  note: cnt
  note: deg motor
  In1 : Inport
  Constant3 : Constant  Value=360
  Product3 : Product  Inputs=*/
  Product4 : Product  Inputs=**
  Product5 : Product  Inputs=*/
  Out1 : Outport
  wires:
  In1/1 -> Product4/1
  [cpt_sus] -> Product3/2
  Product4/1 -> Product5/1
  [N_sus] -> Product5/2
  Product5/1 -> Out1/1
  Product3/1 -> Product4/2
  Constant3/1 -> Product3/1

== system Katex_FullCar_R2017b_V03/DGIST/Subsystem3 ==
  In1 : Inport
  Product : Product  Inputs=*/
  rpm2rad2 : Gain  Gain=2*pi/60
  Out1 : Outport
  wires:
  Product/1 -> Out1/1  "Load (rad/s)"
  In1/1 -> rpm2rad2/1  "rpm"
  [N_sus] -> Product/2
  rpm2rad2/1 -> Product/1  "rad/s"

== system Katex_FullCar_R2017b_V03/DGIST/Subsystem4 ==
  note: Motor Nm
  note: mNm
  note: A
  note: mNm/A
  In1 : Inport
  Divide4 : Product  Inputs=**
  Divide5 : Product  Inputs=**
  Torque Constant3 : Gain  Gain=0.001
  mA2A1 : Gain  Gain=0.001
  Out1 : Outport
  wires:
  Torque Constant3/1 -> Divide4/1
  mA2A1/1 -> Divide5/2
  [sus_Torque_constant] -> Divide5/1
  Divide5/1 -> Torque Constant3/1
  [N_sus] -> Divide4/2
  Divide4/1 -> Out1/1
  In1/1 -> mA2A1/1

== system Katex_FullCar_R2017b_V03/DGIST/Subsystem5 ==
  note: mNm/A
  note: Motor Nm
  note: A
  In1 : Inport
  Divide : Product  Inputs=**
  Divide3 : Product  Inputs=**
  Torque Constant2 : Gain  Gain=0.001
  mA2A2 : Gain  Gain=0.001
  Out1 : Outport
  wires:
  [N_str] -> Divide3/2
  Torque Constant2/1 -> Divide3/1
  Divide/1 -> Torque Constant2/1
  [str_Torque_constant] -> Divide/1
  Divide3/1 -> Out1/1  "Load Nm"
  mA2A2/1 -> Divide/2
  In1/1 -> mA2A2/1

== system Katex_FullCar_R2017b_V03/DGIST/Subsystem6 ==
  note: deg motor
  note: cnt
  note: deg load
  In1 : Inport
  Constant2 : Constant  Value=360
  Product : Product  Inputs=*/
  Product1 : Product  Inputs=**
  Product2 : Product  Inputs=*/
  Out1 : Outport
  wires:
  Constant2/1 -> Product/1
  Product2/1 -> Out1/1
  [cpt_str] -> Product/2
  [N_str] -> Product2/2
  Product/1 -> Product1/2
  In1/1 -> Product1/1
  Product1/1 -> Product2/1

== system Katex_FullCar_R2017b_V03/DGIST/Subsystem7 ==
  In : Inport
  LPF : Subsystem
  Out : Outport
  wires:
  In/1 -> LPF/1(In)
  LPF/1(Out) -> Out/1

== system Katex_FullCar_R2017b_V03/DGIST/Subsystem8 ==
  In : Inport
  LPF : Subsystem
  Out : Outport
  wires:
  In/1 -> LPF/1(In)
  LPF/1(Out) -> Out/1

== system Katex_FullCar_R2017b_V03/DGIST/Subsystem9 ==
  In : Inport
  LPF : Subsystem
  Out : Outport
  wires:
  In/1 -> LPF/1(In)
  LPF/1(Out) -> Out/1

== system Katex_FullCar_R2017b_V03/DGIST/_High_Level_Ctrl ==
  note: Vx,YawRate Ref Scope(2X1)
  note: rad/s
  note: Torque Mode면 Load Vel을 motor로 바꿔서  input으로
      | Pos,Vel mode면Output이 Vel,Pos를 Motor로 바로 바꾸는 알고리즘
  note: Drive_Ref 4X1
  note: 전륜 구동만, 후륜은 v_x estimation으로 사용
      |
      | Input : v_x, gamma
      | output : 전륜 모터 각속도, 전륜 steering angle
  note: Design Todo List 및 Block에 대한 큰 설명
      |
      | Input
      | - Chassis 4자유도 reference (Vx_ref , YawRate_ref, RollRate_ref, PitchRate)
      |
      | Output
      | - Driving Motor Trajectory (Velocity)
      | - Steering Motor Trajectory (Position)
      | - Suspension Motor Trajectory (Velocity , Position)
      |
      | Block에 대한 큰 설명
  note: 4륜 구동
      |
      | Input : v_x, gamma
      | output : 모터 각속도, steering angle
  note: Suspension Orientation DOB Control
      |
      | Input : Roll,Pitch
      | output : Suspension Load 각속도(rad/s)
  note: Steer_Ref 4X1
  note: Drive_Ref 4X1
  note: Steer_Ref 4X1
  note: rad
  note: Suspension Position Mode
      |
      | Input : Roll,Pitch
      | output : Suspension Load 각도 (deg)
  note: deg
  note: Vx,YawRate Ref Scope(2X1)
  note: deg/s
  note: m/s
  Chassis_FB_ctrl : Subsystem
      mask Display: disp('Chassis_FB_ctrl');
  Chassis_FF_ctrl : Subsystem
      mask Display: disp('Chassis_FF_ctrl');
  Constant : Constant  Value=180/pi
  Constant1 : Constant  Value=locklim_sus-5
  Demux2 : Demux  Outputs=2
  Demux3 : Demux  Outputs=2
  Divide : Product  Inputs=**
  Gain : Gain  Gain=-1
  If Action Subsystem1 : Subsystem  TreatAsAtomicUnit=on
  If Action Subsystem5 : Subsystem  TreatAsAtomicUnit=on
  If1 : If  IfExpression=u1 == 0  ElseIfExpressions=u1 == 1
  Merge1 : Merge
  Merge2 : Merge
  Merge3 : Merge
  Orientation_Pos_Ctrl : Subsystem
      mask Display: disp('Orientation_Ctrl');
  Orientation_Vel_Ctrl : Subsystem  Commented=on
      mask Display: disp('Orientation_Ctrl');
  Saturation Dynamic : sl_discontinuities/Saturation Dynamic  OutMin=[]  OutMax=[]  OutDataTypeStr=Inherit: Same as second input  OutDataType=fixdt(1, 16)  OutScaling=2^-10  DoSatur=off
  Dri_Load_Vel_Ref : Outport
  Str_Load_Vel_Ref : Outport  Port=2
  Out1 : Outport  Port=3
  tag scope: Body_Pitch_deg_scope=global, Body_Roll_deg_scope=global, Body_Yawrate_degps_scope=global, Body_vx_mps_scope=global
  wires:
  Chassis_FF_ctrl/1(FF_DriveVel_ref) -> If Action Subsystem5/1(In1)
  Chassis_FF_ctrl/2(FF_SteerPos_ref) -> If Action Subsystem5/2(In2)
  If1/1 -> If Action Subsystem5/Action
  Chassis_FB_ctrl/1(FF_DriveVel_ref) -> If Action Subsystem1/1(In1)
  Chassis_FB_ctrl/2(FF_SteerPos_ref) -> If Action Subsystem1/2(In2)
  [Chassis_FB_OnOff] -> If1/1
  If1/2 -> If Action Subsystem1/Action
  If Action Subsystem5/1(Out1) -> Merge2/1
  If Action Subsystem1/1(Out1) -> Merge2/2
  If Action Subsystem5/2(Out2) -> Merge1/1
  If Action Subsystem1/2(Out2) -> Merge1/2
  Merge2/1 -> Dri_Load_Vel_Ref/1
  Merge1/1 -> Divide/1
  Constant/1 -> Divide/2
  Divide/1 -> Saturation Dynamic/2
  Constant1/1 -> Gain/1, Saturation Dynamic/1
  Gain/1 -> Saturation Dynamic/3
  Merge3/1 -> Demux2/1
  Orientation_Pos_Ctrl/1(Out1) -> Demux3/1
  Demux2/1 -> [Body_vx_mps_scope]
  Demux2/2 -> [Body_Yawrate_degps_scope]
  Demux3/1 -> [Body_Roll_deg_scope]
  Demux3/2 -> [Body_Pitch_deg_scope]
  Chassis_FF_ctrl/3(Body_ref_scope) -> If Action Subsystem5/3(In3)
  Chassis_FB_ctrl/3(Body_ref_scope) -> If Action Subsystem1/3(In3)
  If Action Subsystem1/3(Out3) -> Merge3/2
  If Action Subsystem5/3(Out3) -> Merge3/1
  Saturation Dynamic/1 -> Str_Load_Vel_Ref/1
  Orientation_Pos_Ctrl/2(Ori_Sus_Load_Pos_Ref) -> Out1/1

== system Katex_FullCar_R2017b_V03/DGIST/_Low_Level_Ctrl ==
  In1 : Inport
  In2 : Inport  Port=2
  In3 : Inport  Port=3
  Driving_Low_Level_Controller : Subsystem
      mask Display: disp('Driving Low Level Controller');
  Steering_Low_Level_Controller : Subsystem
      mask Display: disp('Steering_Low_Level_Controller');
  Suspension_Low_Level_Controller : Subsystem
      mask Display: disp('Suspension Low Level Controller');
  Out1 : Outport
  Out2 : Outport  Port=2
  Out3 : Outport  Port=3
  wires:
  In1/1 -> Driving_Low_Level_Controller/1(In1)
  In2/1 -> Steering_Low_Level_Controller/1(In1)
  Suspension_Low_Level_Controller/1(Out1) -> Out3/1
  Steering_Low_Level_Controller/1(Out1) -> Out2/1
  Driving_Low_Level_Controller/1(Out1) -> Out1/1
  In3/1 -> Suspension_Low_Level_Controller/1(In1)

== system Katex_FullCar_R2017b_V03/DGIST/_Reference_Generator ==
  note: output
      |
      | Vx
      | gamma
      | RollRate
      | PitchRate
  Constant : Constant  Value=0
  Demux : Demux
  If Action Subsystem1 : Subsystem  TreatAsAtomicUnit=on
  If Action Subsystem2 : Subsystem  TreatAsAtomicUnit=on
  If Action Subsystem3 : Subsystem  TreatAsAtomicUnit=on
  If Action Subsystem4 : Subsystem  TreatAsAtomicUnit=on
  If2 : If  IfExpression=u1 == 1  ElseIfExpressions=u1 == 2,u1 == 3
  Merge2 : Merge  Inputs=4
  Mux : Mux
  Orientation Profile : Subsystem
      mask Display: disp('Orientation Profile');
  Scope : Scope
      settings: DataLoggingVariableName=ScopeData2
  Slalom Profile : Subsystem
      mask Display: disp('Slalom Profile');
  Straight Profile : Subsystem
      mask Display: disp('Straight Profile');
  tag scope: Body_PitchRate_ref=global, Body_RollRate_ref=global, Body_Vx_ref=global, Body_YawRate_ref=global
  wires:
  [Local_Time] -> Scope/1
  [Scenario_cmd] -> If2/1
  If2/1 -> If Action Subsystem4/Action
  If2/2 -> If Action Subsystem1/Action
  If2/3 -> If Action Subsystem2/Action
  If2/4 -> If Action Subsystem3/Action
  Straight Profile/1(Ref1_Output) -> If Action Subsystem4/1(In1)
  Constant/1 -> Mux/4, Mux/3, Mux/2, Mux/1
  Mux/1 -> If Action Subsystem3/1(In1)
  Slalom Profile/1(Ref2_Output) -> If Action Subsystem1/1(In1)
  Orientation Profile/1(Ref3_Output) -> If Action Subsystem2/1(In1)
  If Action Subsystem4/1(Out1) -> Merge2/1
  If Action Subsystem1/1(Out1) -> Merge2/2
  If Action Subsystem2/1(Out1) -> Merge2/3
  If Action Subsystem3/1(Out1) -> Merge2/4
  Merge2/1 -> Demux/1
  Demux/1 -> [Body_Vx_ref]
  Demux/2 -> [Body_YawRate_ref]
  Demux/3 -> [Body_RollRate_ref]
  Demux/4 -> [Body_PitchRate_ref]

== system Katex_FullCar_R2017b_V03/Locomotion/Branch ==
  drv_velref_mps : Inport
  drv_tqref_Nm : Inport  Port=2
  str_angref_deg : Inport  Port=3
  str_tqref_Nm : Inport  Port=4
  sus_angref_deg : Inport  Port=5
  sus_tqref_Nm : Inport  Port=6
  Bus Creator{,1..3} (4 alike) : BusCreator  Inputs=6
  Demux{,1..5} (6 alike) : Demux
  Gain{,1..23} (24 alike) : Gain
  Scope : Scope  NumInputPorts=4
      settings: ActiveDisplayYMinimum=-1  ActiveDisplayYMaximum=1  DataLoggingVariableName=ScopeData80
  FL : Outport  VectorParamsAs1DForOutWhenUnconnected=off
  FR : Outport  Port=2  VectorParamsAs1DForOutWhenUnconnected=off
  RL : Outport  Port=3  VectorParamsAs1DForOutWhenUnconnected=off
  RR : Outport  Port=4  VectorParamsAs1DForOutWhenUnconnected=off
  wires:
  Gain9/1 -> Bus Creator2/2  "RLdrv_tqref_pct"
  Gain15/1 -> Scope/3, Bus Creator2/5  "RLsus_angref_deg"
  Gain10/1 -> Bus Creator3/3  "RRstr_angref_deg"
  Gain11/1 -> Bus Creator2/3  "RLstr_angref_deg"
  Gain20/1 -> Bus Creator1/6  "FRsus_tqref_pct"
  Gain5/1 -> Bus Creator/3  "FLstr_angref_deg"
  Gain3/1 -> Bus Creator/1  "FLdrv_velref_mps"
  Gain23/1 -> Bus Creator2/6  "RLsus_tqref_pct"
  Gain19/1 -> Bus Creator/4  "FLstr_tqref_pct"
  Gain/1 -> Bus Creator1/1  "FRdrv_velref_mps"
  Gain4/1 -> Bus Creator/2  "FLdrv_tqref_pct"
  Gain21/1 -> Bus Creator/6  "FLsus_tqref_pct"
  Gain1/1 -> Bus Creator1/2  "FRdrv_tqref_pct"
  Gain14/1 -> Scope/4, Bus Creator3/5  "RRsus_angref_deg"
  Gain16/1 -> Bus Creator3/4  "RRstr_tqref_pct"
  Gain13/1 -> Bus Creator/5, Scope/1  "FLsus_angref_deg"
  Gain8/1 -> Bus Creator3/2  "RRdrv_tqref_pct"
  Gain12/1 -> Bus Creator1/5, Scope/2  "FRsus_angref_deg"
  Gain6/1 -> Bus Creator3/1  "RRdrv_velref_mps"
  Gain22/1 -> Bus Creator3/6  "RRsus_tqref_pct"
  Gain7/1 -> Bus Creator2/1  "RLdrv_velref_mps"
  Gain17/1 -> Bus Creator2/4  "RLstr_tqref_pct"
  Bus Creator/1 -> FL/1  "FL"
  Bus Creator1/1 -> FR/1  "FR"
  Bus Creator2/1 -> RL/1  "RL"
  Bus Creator3/1 -> RR/1  "RR"
  Gain18/1 -> Bus Creator1/4  "FRstr_tqref_pct"
  Gain2/1 -> Bus Creator1/3  "FRstr_angref_deg"
  Demux/1 -> Gain5/1
  Demux/2 -> Gain2/1
  Demux/3 -> Gain11/1
  Demux/4 -> Gain10/1
  str_angref_deg/1 -> Demux/1
  drv_velref_mps/1 -> Demux1/1
  Demux1/1 -> Gain3/1
  Demux1/2 -> Gain/1
  Demux1/3 -> Gain7/1
  Demux1/4 -> Gain6/1
  Demux2/2 -> Gain1/1
  Demux2/1 -> Gain4/1
  Demux2/3 -> Gain9/1
  Demux2/4 -> Gain8/1
  drv_tqref_Nm/1 -> Demux2/1
  Demux3/1 -> Gain19/1
  Demux3/3 -> Gain17/1
  Demux3/4 -> Gain16/1
  Demux3/2 -> Gain18/1
  str_tqref_Nm/1 -> Demux3/1
  Demux4/1 -> Gain13/1
  Demux4/2 -> Gain12/1
  Demux4/3 -> Gain15/1
  Demux4/4 -> Gain14/1
  sus_angref_deg/1 -> Demux4/1
  Demux5/1 -> Gain21/1
  Demux5/2 -> Gain20/1
  Demux5/3 -> Gain23/1
  Demux5/4 -> Gain22/1
  sus_tqref_Nm/1 -> Demux5/1

== system Katex_FullCar_R2017b_V03/Locomotion/Conditioning ==
  note: [1] Front-wheel (전륜)
      | [2] In-phase (동상)
      | [3] Anti-phase (역상)
      | [4] Zero-turn
  note: [0] All synchronize
      | [1] Only FL
      | [2] Only FR
      | [3] Only RL
      | [4] Only RR
  CMD_DRV_VELOCITY : Inport
  CMD_DRV_TORQUE : Inport  Port=2
  CMD_STR_ANGLE : Inport  Port=3
  CMD_STR_TORQUE : Inport  Port=4
  CMD_SUS_ANGLE : Inport  Port=5
  CMD_SUS_TORQUE : Inport  Port=6
  Constant : Constant  Value=-2.68
  Driving mode : Subsystem
  Drv_LPF : Subsystem
  Drv_LPF1 : Subsystem
  Drv_LPF2 : Subsystem
  Drv_LPF3 : Subsystem
  Mux : Mux
  Point_Round1 : Subsystem
  Point_Round3 : Subsystem
  Point_Round4 : Subsystem
  STR_LPF_cutoff : Constant  SampleTime=Ts
  STR_LPF_cutoff1 : Constant  SampleTime=Ts
  Steering mode : Subsystem
  Str_LPF : Subsystem
  Sus_LPF : Subsystem
  Sus_Saturation : Saturate  UpperLimit=40  LowerLimit=-40
  Suspension mode : Subsystem
  drv_LPF_cutoff : Constant  Value=3  SampleTime=Ts
  drv_LPF_cutoff1 : Constant  SampleTime=Ts
  drv_tq_saturation : Saturate  UpperLimit=300  LowerLimit=-300
  roundN1 : Constant  Value=roundN
  roundN3 : Constant  Value=roundN
  roundN4 : Constant  Value=roundN
  str_LPF_cutoff : Constant  Value=3  SampleTime=Ts
  str_mode : Constant  Value=3
  str_tq_saturation : Saturate  UpperLimit=100  LowerLimit=-100
  sus_LPF_cutoff : Constant  Value=3  SampleTime=Ts
  sus_mode : Constant  Value=0
  sus_tq_saturation : Saturate  UpperLimit=100  LowerLimit=-100
  Drv_velocity : Outport  VectorParamsAs1DForOutWhenUnconnected=off
  Drv_torque : Outport  Port=2  VectorParamsAs1DForOutWhenUnconnected=off
  Str_angle : Outport  Port=3  VectorParamsAs1DForOutWhenUnconnected=off
  Str_torque : Outport  Port=4  VectorParamsAs1DForOutWhenUnconnected=off
  Sus_angle : Outport  Port=5  VectorParamsAs1DForOutWhenUnconnected=off
  Sus_torque : Outport  Port=6  VectorParamsAs1DForOutWhenUnconnected=off
  wires:
  str_mode/1 -> Driving mode/2(mode), Steering mode/1(mode)
  CMD_SUS_ANGLE/1 -> Suspension mode/2(cmd)
  Suspension mode/1(cmd_out) -> Sus_Saturation/1
  CMD_DRV_VELOCITY/1 -> Driving mode/1(cmd)
  Steering mode/1(cmd_out) -> Str_LPF/1(In)
  Drv_LPF1/1(Out) -> Drv_torque/1
  Sus_Saturation/1 -> Sus_LPF/1(In)
  CMD_DRV_TORQUE/1 -> drv_tq_saturation/1
  CMD_STR_ANGLE/1 -> Steering mode/2(cmd)
  Driving mode/1(cmd_out) -> Drv_LPF/1(In)
  Drv_LPF3/1(Out) -> Sus_torque/1
  Sus_LPF/1(Out) -> Point_Round4/1(u)
  Str_LPF/1(Out) -> Point_Round3/1(u)
  sus_LPF_cutoff/1 -> Sus_LPF/2(fc)
  roundN3/1 -> Point_Round3/2(N)
  Drv_LPF/1(Out) -> Point_Round1/1(u)
  str_LPF_cutoff/1 -> Str_LPF/2(fc)
  roundN1/1 -> Point_Round1/2(N)
  drv_LPF_cutoff/1 -> Drv_LPF/2(fc)
  roundN4/1 -> Point_Round4/2(N)
  Point_Round1/1(y) -> Drv_velocity/1  "drv_velref_mps"
  Point_Round3/1(y) -> Str_angle/1  "str_angref_deg"
  Point_Round4/1(y) -> Sus_angle/1  "sus_angref_deg"
  drv_tq_saturation/1 -> Drv_LPF1/1(In)
  sus_mode/1 -> Suspension mode/1(mode)
  drv_LPF_cutoff1/1 -> Drv_LPF1/2(fc)
  CMD_STR_TORQUE/1 -> str_tq_saturation/1
  str_tq_saturation/1 -> Drv_LPF2/1(In)
  STR_LPF_cutoff/1 -> Drv_LPF2/2(fc)
  sus_tq_saturation/1 -> Drv_LPF3/1(In)
  STR_LPF_cutoff1/1 -> Drv_LPF3/2(fc)
  Drv_LPF2/1(Out) -> Str_torque/1
  CMD_SUS_TORQUE/1 -> sus_tq_saturation/1
  Constant/1 -> Mux/4, Mux/3, Mux/2, Mux/1

== system Katex_FullCar_R2017b_V03/Locomotion/If Action Subsystem ==
  In1 : Inport
  Action Port : ActionPort  ActionPortLabel=if(u1 == 1)
  CMD_DRV_VELOCITY : Outport
  wires:
  In1/1 -> CMD_DRV_VELOCITY/1

== system Katex_FullCar_R2017b_V03/Locomotion/If Action Subsystem1 ==
  Driving : Inport
  Action Port : ActionPort  ActionPortLabel=elseif(u1 == 2)
  CMD_DRV_VELOCITY : Outport
  wires:
  Driving/1 -> CMD_DRV_VELOCITY/1

== system Katex_FullCar_R2017b_V03/Locomotion/If Action Subsystem2 ==
  In1 : Inport
  Action Port : ActionPort  ActionPortLabel=if(u1 == 0||u1==1)
  CMD_DRV_VELOCITY : Outport
  wires:
  In1/1 -> CMD_DRV_VELOCITY/1

== system Katex_FullCar_R2017b_V03/Locomotion/If Action Subsystem3 ==
  Driving : Inport
  Action Port : ActionPort  ActionPortLabel=elseif(u1 == 2)
  CMD_DRV_VELOCITY : Outport
  wires:
  Driving/1 -> CMD_DRV_VELOCITY/1

== system Katex_FullCar_R2017b_V03/Locomotion/If Action Subsystem4 ==
  Suspension : Inport
  Action Port : ActionPort  ActionPortLabel=if(u1 == 0||u1==1)
  CMD_DRV_VELOCITY : Outport
  wires:
  Suspension/1 -> CMD_DRV_VELOCITY/1

== system Katex_FullCar_R2017b_V03/Locomotion/If Action Subsystem5 ==
  Driving : Inport
  Action Port : ActionPort  ActionPortLabel=elseif(u1 == 2)
  CMD_DRV_VELOCITY : Outport
  wires:
  Driving/1 -> CMD_DRV_VELOCITY/1
